simulink model "Accelerator"  (R2019a)
settings: Solver=FixedStepAuto  StartTime=0.0  StopTime=4  FixedStep=step  RelTol=1e-3
model workspace (MAT data in the model file):
  a = Simulink.Signal
  a.DataType = 'double'
  a.DocUnits = 'rad/S^2'
  a.Dimensions = 1
  a.DimensionsMode = 'Fixed'
  a.Complexity = 'real'
  a.SampleTime = -1
  a.SamplingMode = 'auto'
  a.InitialValue = '0'
  d = Simulink.Signal
  d.DataType = 'double'
  d.DocUnits = 'rad'
  d.Dimensions = 1
  d.DimensionsMode = 'Fixed'
  d.Complexity = 'real'
  d.SampleTime = -1
  d.SamplingMode = 'auto'
  d.InitialValue = '0'
  j = Simulink.Signal
  j.DataType = 'double'
  j.DocUnits = 'rad/S^3'
  j.Dimensions = 1
  j.DimensionsMode = 'Fixed'
  j.Complexity = 'real'
  j.SampleTime = -1
  j.SamplingMode = 'auto'
  j.InitialValue = '1000'
  step = 0.001
  t_AASearch = Simulink.Signal
  t_AASearch.Description = 'This variable is the searching tolernece for DS.'
  t_AASearch.DataType = 'double'
  t_AASearch.DocUnits = 'm'
  t_AASearch.Dimensions = 1
  t_AASearch.DimensionsMode = 'auto'
  t_AASearch.Complexity = 'real'
  t_AASearch.SampleTime = -1
  t_AASearch.SamplingMode = 'auto'
  t_AASearch.InitialValue = '0.001'
  v = Simulink.Signal
  v.DataType = 'double'
  v.Dimensions = 1
  v.DimensionsMode = 'auto'
  v.Complexity = 'real'
  v.SampleTime = -1
  v.SamplingMode = 'auto'
  v.InitialValue = '0'
settings Model: OrderedModelArguments=off  Creator=EiLit  LastModifiedBy=EiLit
settings DataIOCC: ReturnWorkspaceOutputs=off
settings DebuggingCC: ReadBeforeWriteMsg=EnableAllAsWarning  WriteAfterWriteMsg=EnableAllAsWarning  WriteAfterReadMsg=EnableAllAsWarning  ArithmeticOperatorsInVariantConditions=warning

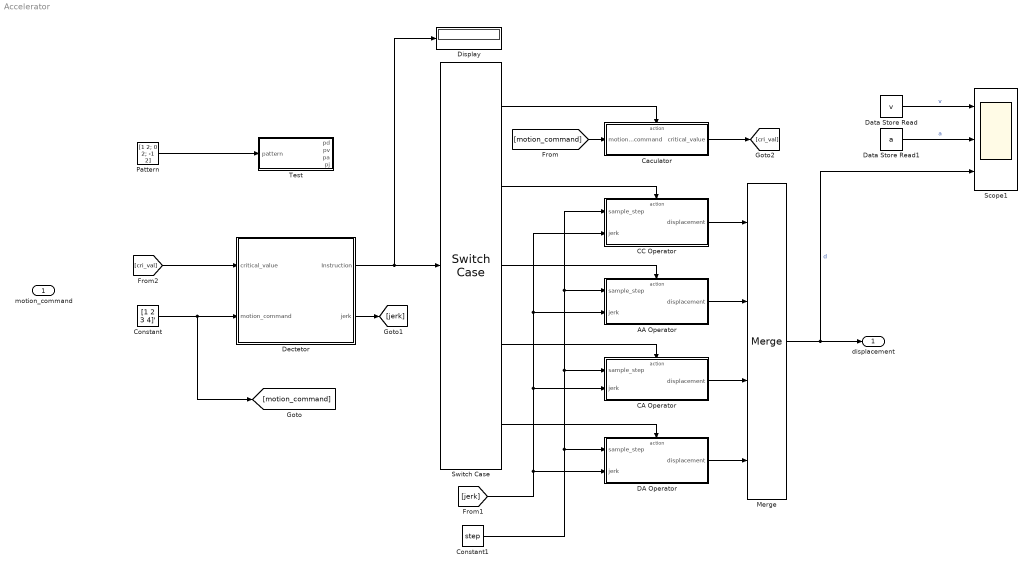
== system Accelerator ==
  motion_command : Inport
  AA Operator : Subsystem  TreatAsAtomicUnit=on
  CA Operator : Subsystem  TreatAsAtomicUnit=on
  CC Operator : Subsystem  TreatAsAtomicUnit=on
  Caculator : Subsystem  TreatAsAtomicUnit=on
  Constant : Constant  Value=[1 2 3 4]'
  Constant1 : Constant  Value=step
  DA Operator : Subsystem  TreatAsAtomicUnit=on
  Data Store Read : DataStoreRead  DataStoreName=v
  Data Store Read1 : DataStoreRead  DataStoreName=a
  Dectetor : Subsystem
  Display : Display
  Merge : Merge  Inputs=4  InitialOutput=[0]
  Pattern : Constant  Value=[1 2; 0 2; -1 2]  VectorParams1D=off
  Scope1 : Scope  NumInputPorts=3
  Switch Case : SwitchCase  CaseConditions={0,1,2,3,4}  ShowDefaultCase=off
  Test : Subsystem
  displacement : Outport
  wires:
  Dectetor/1(Instruction) -> Switch Case/1, Display/1
  Switch Case/1 -> Caculator/Action
  Switch Case/2 -> CC Operator/Action
  Switch Case/3 -> AA Operator/Action
  Switch Case/4 -> CA Operator/Action
  Switch Case/5 -> DA Operator/Action
  DA Operator/1(displacement) -> Merge/4
  CC Operator/1(displacement) -> Merge/1
  AA Operator/1(displacement) -> Merge/2
  CA Operator/1(displacement) -> Merge/3
  Merge/1 -> Scope1/3, displacement/1  "d"
  Constant/1 -> Dectetor/2(motion_command), [motion_command]
  Data Store Read/1 -> Scope1/1  "v"
  Data Store Read1/1 -> Scope1/2  "a"
  [motion_command] -> Caculator/1(motion_command)
  Constant1/1 -> DA Operator/1(sample_step), AA Operator/1(sample_step), CC Operator/1(sample_step), CA Operator/1(sample_step)
  Dectetor/2(jerk) -> [jerk]
  Caculator/1(critical_value) -> [cri_val]
  [cri_val] -> Dectetor/1(critical_value)
  [jerk] -> CA Operator/2(jerk), CC Operator/2(jerk), AA Operator/2(jerk), DA Operator/2(jerk)
  Pattern/1 -> Test/1(pattern)

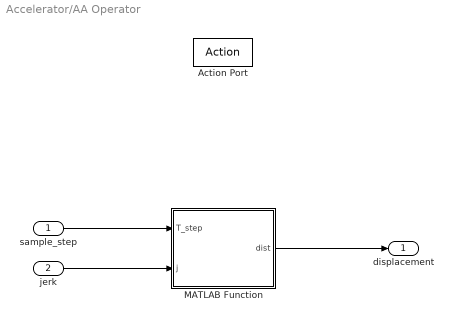
== system Accelerator/AA Operator ==
  sample_step : Inport
  jerk : Inport  Port=2
  Action Port : ActionPort  ActionPortLabel=case [ 2 ]:
  MATLAB Function : MATLAB Function  TreatAsAtomicUnit=on
  displacement : Outport  PortDimensions=1
  wires:
  sample_step/1 -> MATLAB Function/1(T_step)
  MATLAB Function/1(dist) -> displacement/1
  jerk/1 -> MATLAB Function/2(j)

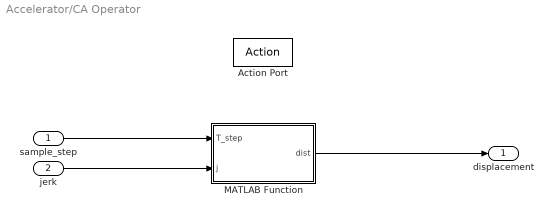
== system Accelerator/CA Operator ==
  sample_step : Inport
  jerk : Inport  Port=2
  Action Port : ActionPort  ActionPortLabel=case [ 3 ]:
  MATLAB Function : MATLAB Function  TreatAsAtomicUnit=on
  displacement : Outport
  wires:
  sample_step/1 -> MATLAB Function/1(T_step)
  MATLAB Function/1(dist) -> displacement/1
  jerk/1 -> MATLAB Function/2(j)

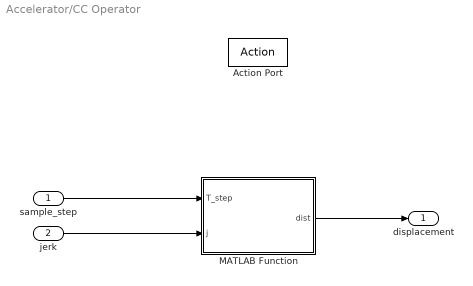
== system Accelerator/CC Operator ==
  sample_step : Inport
  jerk : Inport  Port=2
  Action Port : ActionPort  ActionPortLabel=case [ 1 ]:
  MATLAB Function : MATLAB Function  TreatAsAtomicUnit=on
  displacement : Outport
  wires:
  MATLAB Function/1(dist) -> displacement/1
  jerk/1 -> MATLAB Function/2(j)
  sample_step/1 -> MATLAB Function/1(T_step)

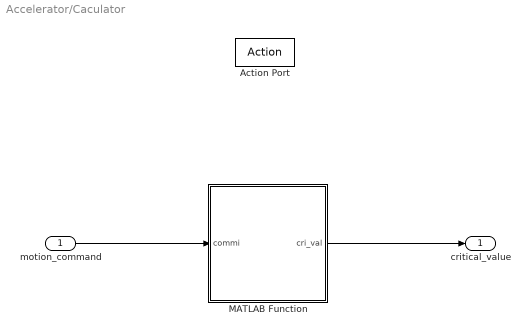
== system Accelerator/Caculator ==
  motion_command : Inport
  Action Port : ActionPort  ActionPortLabel=case [ 0 ]:
  MATLAB Function : MATLAB Function  TreatAsAtomicUnit=on
  critical_value : Outport
  wires:
  motion_command/1 -> MATLAB Function/1(commi)
  MATLAB Function/1(cri_val) -> critical_value/1

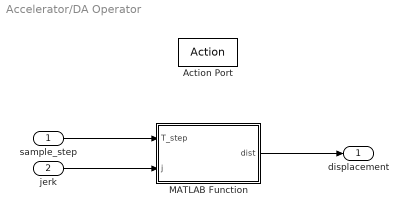
== system Accelerator/DA Operator ==
  sample_step : Inport
  jerk : Inport  Port=2
  Action Port : ActionPort  ActionPortLabel=case [ 4 ]:
  MATLAB Function : MATLAB Function  TreatAsAtomicUnit=on
  displacement : Outport
  wires:
  sample_step/1 -> MATLAB Function/1(T_step)
  MATLAB Function/1(dist) -> displacement/1
  jerk/1 -> MATLAB Function/2(j)

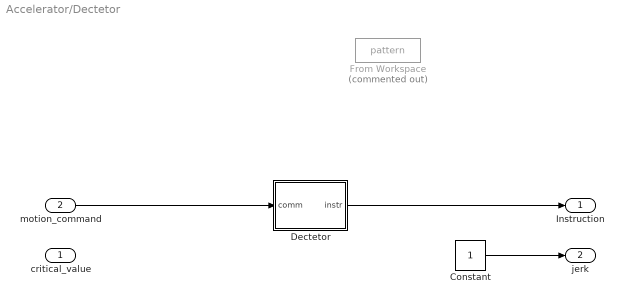
== system Accelerator/Dectetor ==
  critical_value : Inport
  motion_command : Inport  Port=2
  Constant : Constant
  Dectetor : MATLAB Function  TreatAsAtomicUnit=on
  From Workspace : FromWorkspace  Commented=on  VariableName=pattern  SampleTime=0
  Instruction : Outport
  jerk : Outport  Port=2
  wires:
  motion_command/1 -> Dectetor/1(comm)
  Dectetor/1(instr) -> Instruction/1
  Constant/1 -> jerk/1

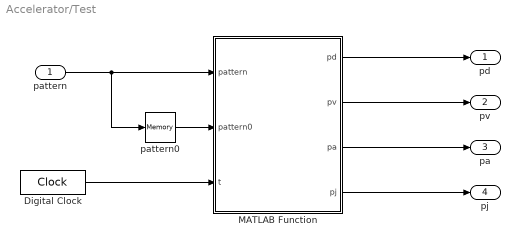
== system Accelerator/Test ==
  pattern : Inport
  Digital Clock : DigitalClock
  MATLAB Function : MATLAB Function  TreatAsAtomicUnit=on
  pattern0 : Memory
  pd : Outport
  pv : Outport  Port=2
  pa : Outport  Port=3
  pj : Outport  Port=4
  wires:
  pattern/1 -> MATLAB Function/1(pattern), pattern0/1
  MATLAB Function/1(pd) -> pd/1
  pattern0/1 -> MATLAB Function/2(pattern0)
  Digital Clock/1 -> MATLAB Function/3(t)
  MATLAB Function/4(pj) -> pj/1
  MATLAB Function/3(pa) -> pa/1
  MATLAB Function/2(pv) -> pv/1

== matlab function Accelerator/Dectetor/Dectetor ==
  data: comm input; instr output
function instr = fcn(comm)

instr = 1;

== matlab function Accelerator/CC Operator/MATLAB Function ==
  data: T_step input; dist output; v data_store_memory; d data_store_memory; a data_store_memory; j input
function dist = fcn(T_step,j)
global d v a
a = 0;
d = d + v*T_step;
dist = d;

== matlab function Accelerator/AA Operator/MATLAB Function ==
  data: T_step input; dist output; d data_store_memory; v data_store_memory; a data_store_memory; j input
function dist = fcn(T_step,j)
global d v a
a = a + j*T_step;
v = v + a*T_step + 1/2*j*T_step^2;
d = d + v*T_step + 1/2*a*T_step^2 + 1/6*j*T_step^3;
dist = d;

== matlab function Accelerator/CA Operator/MATLAB Function ==
  data: T_step input; dist output; d data_store_memory; v data_store_memory; a data_store_memory; j input
function dist = fcn(T_step,j)
global d v a
v = v + a*T_step;
d = d + v*T_step + 1/2*a*T_step^2;
dist = d;

== matlab function Accelerator/DA Operator/MATLAB Function ==
  data: T_step input; dist output; d data_store_memory; v data_store_memory; a data_store_memory; j input
function dist = fcn(T_step,j)
global d v a
a = a - j*T_step;
v = v + a*T_step - 1/2*j*T_step^2;
d = d + v*T_step + 1/2*a*T_step^2 - 1/6*j*T_step^3;
dist = d;

== matlab function Accelerator/Caculator/MATLAB Function ==
  data: commi input; d data_store_memory; v data_store_memory; a data_store_memory; cri_val output; t_AASearch data_store_memory
function cri_val = fcn(commi)
%% Preprocess
global d v a t_AASearch
% Reset the displacement
d = 0;

% Deal with the direction.
comm = commi;
if commi(1) < 0
    comm = -abs(comm);
end

%% Deal with the pre-acceleration process
% This pre phase should be dealed with at the first step, as it is fixed.
pre_cr = Pre_Acc(comm, d, v, a);

%% Velocity Shortage Determination
% The difference judgement is used, as the correction need the jerk.
% Compute the modified command.
comm_velmod = VelS_ComCal(comm,pre_cr);

%% 1st Standard Process Calculation
% This is to calculate the critical values for the standard
% process. Based on these values, further determination can be made.
[d_cr, v_cr, a_cr, t_cr] = Std_PRO_cr(comm_velmod, pre_cr);    
    
%% Displacement Shortage Determination
DS_flag = DisS_Judge(d_cr,comm);

if DS_flag
    [Ind,ds_cr,vs_cr,as_cr,ts_cr] = DisS_CJ(d_cr,comm_velmod,pre_cr);
    switch Ind
        case 1          %The DS can't be made up
            d_cr = ds_cr;
            v_cr = vs_cr;
            a_cr = as_cr;
            t_cr = ts_cr;
        case 2          %The DS can be made up by modifing the CA step
            [d_cr, v_cr, a_cr, t_cr] = DisS_CAModiCal(d_cr,v_cr,t_cr,comm_velmod,pre_cr);
        case 3          %The DS can be made up by changing the acceleration
            dis_comm = comm_velmod;
            if length(comm_velmod) < 5          % If is feedrate shortage
                dis_comm(2) = dis_comm(2) - min(v_cr(3)-v_cr(2), v_cr(7)-v_cr(6));
            end
            [d_cr, v_cr, a_cr, t_cr] = DisS_AAModiCal(dis_comm, pre_cr, t_AASearch);
    end
end

%% Postprocess
cri_val = [d_cr v_cr a_cr t_cr];
end

== matlab function Accelerator/Test/MATLAB Function ==
  data: pattern input; pd output; pattern0 input; pv output; pa output; pj output; d data_store_memory; v data_store_memory; a data_store_memory; t input
function [pd, pv, pa, pj] = fcn(pattern, pattern0, t)
global d v a

if pattern ~= pattern0
    d0 = d;
    v0 = v;
    a0 = a;
    t0 = t;
end

[plotData, plotTime] = ProfileGenerator(pattern,d0,v0,a0);

plotTime = plotTime + t0;

pd = plotData(1,plotTime == t);
pv = plotData(2,plotTime == t);
pa = plotData(3,plotTime == t);
pj = plotData(4,plotTime == t);
